simulink model "InverseDynamicsController"  (R2022a)
settings: Solver=VariableStepAuto  StartTime=0.0  StopTime=10.0  RelTol=1e-3
values from neighbouring files (symbols this model uses):
  dt = 0.1    [param.m]    (also in param_10.m; param_7.m)
  F_v = zeros(6,6)    [param.m]    (also in param_10.m; param_7.m)
  K_d = diag([50 50 50 50 50 50])    [param.m]    (also in param_10.m = diag([40 40 40 40 40 40]); param_7.m = diag([40 40 40 40 40 40]))
  K_p = diag([200 200 200 200 200 200])    [param.m]    (also in param_10.m; param_7.m)
  q0 = (ik(T0))'    [param.m]    (also in param_10.m; param_7.m)
settings Model: Creator=niteshkalra  LastModifiedBy=niteshkalra

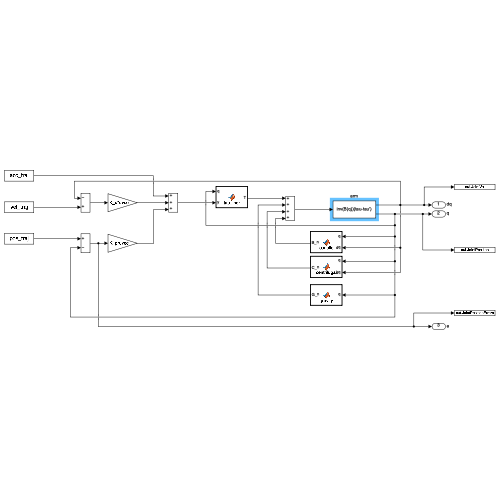
[thumbnail: Simulink's stored preview of the top-level diagram]
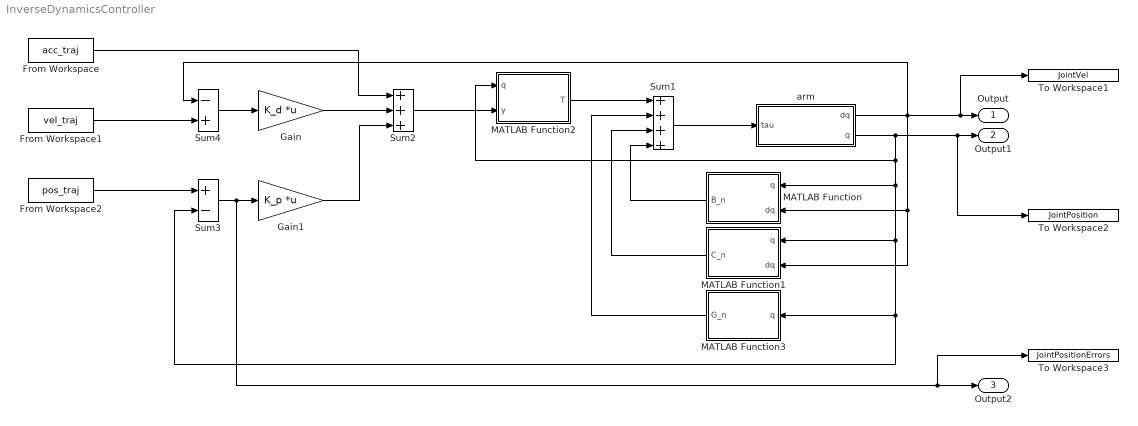
== system InverseDynamicsController ==
  From Workspace : FromWorkspace  VariableName=acc_traj  SampleTime=dt
  From Workspace1 : FromWorkspace  VariableName=vel_traj  SampleTime=dt
  From Workspace2 : FromWorkspace  VariableName=pos_traj  SampleTime=dt
  Gain : Gain  Gain=K_d  Multiplication=Matrix(K*u) (u vector)
  Gain1 : Gain  Gain=K_p  Multiplication=Matrix(K*u) (u vector)
  MATLAB Function : MATLAB Function  TreatAsAtomicUnit=on
  MATLAB Function1 : MATLAB Function  TreatAsAtomicUnit=on
  MATLAB Function2 : MATLAB Function  TreatAsAtomicUnit=on
  MATLAB Function3 : MATLAB Function  TreatAsAtomicUnit=on
  Sum1 : Sum  Inputs=++++
  Sum2 : Sum  Inputs=+++
  Sum3 : Sum  Inputs=+-
  Sum4 : Sum  Inputs=-+
  To Workspace1 : ToWorkspace  VariableName=JointVel  SaveFormat=Timeseries  SampleTime=-1
  To Workspace2 : ToWorkspace  VariableName=JointPosition  SaveFormat=Timeseries  SampleTime=-1
  To Workspace3 : ToWorkspace  VariableName=JointPositionErrors  SaveFormat=Timeseries  SampleTime=-1
  arm : Subsystem
      mask Display: disp('inv(B(q))(tau-tau'')')
  Output : Outport  SignalName=dq
  Output1 : Outport  Port=2  SignalName=q
  Output2 : Outport  Port=3  SignalName=e
  wires:
  MATLAB Function2/1(T) -> Sum1/1
  Sum2/1 -> MATLAB Function2/2(y)
  Gain/1 -> Sum2/2
  Gain1/1 -> Sum2/3
  Sum4/1 -> Gain/1
  From Workspace2/1 -> Sum3/1
  From Workspace/1 -> Sum2/1
  arm/1(dq) -> Sum4/1, MATLAB Function1/2(dq), MATLAB Function/2(dq), To Workspace1/1, Output/1
  arm/2("q ") -> MATLAB Function/1(q), MATLAB Function1/1(q), MATLAB Function3/1(q), Sum3/2, MATLAB Function2/1(q), To Workspace2/1, Output1/1
  Sum3/1 -> To Workspace3/1, Output2/1, Gain1/1
  Sum1/1 -> arm/1(tau)
  MATLAB Function/1(B_n) -> Sum1/4
  MATLAB Function1/1(C_n) -> Sum1/3
  MATLAB Function3/1(G_n) -> Sum1/2
  From Workspace1/1 -> Sum4/2

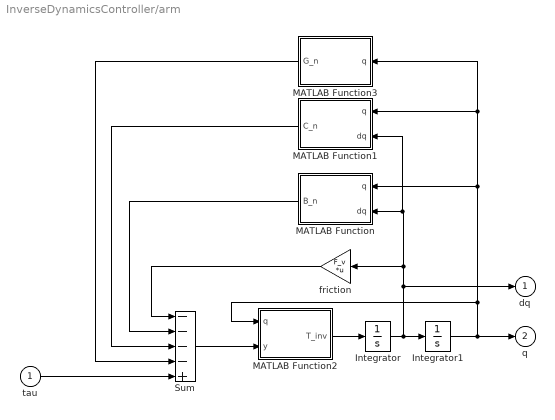
== system InverseDynamicsController/arm ==
  tau : Inport
  Integrator : Integrator  InitialCondition=[0 0 0 0 0 0]'  ZeroCross=off
  Integrator1 : Integrator  InitialCondition=q0  ZeroCross=off
  MATLAB Function : MATLAB Function  TreatAsAtomicUnit=on
  MATLAB Function1 : MATLAB Function  TreatAsAtomicUnit=on
  MATLAB Function2 : MATLAB Function  TreatAsAtomicUnit=on
  MATLAB Function3 : MATLAB Function  TreatAsAtomicUnit=on
  Sum : Sum  Inputs=----+  InputSameDT=on  SaturateOnIntegerOverflow=on  OutDataTypeStr=Inherit: Same as first input
  friction : Gain  Gain=F_v  Multiplication=Matrix(K*u)  SaturateOnIntegerOverflow=on  OutDataTypeStr=Inherit: Same as input  ParamDataTypeStr=Inherit: Same as input
      mask Display: disp('F_v')
  dq : Outport  InitialOutput=0
  "q " : Outport  Port=2  InitialOutput=0
  wires:
  tau/1 -> Sum/5
  Integrator1/1 -> MATLAB Function3/1(q), MATLAB Function1/1(q), MATLAB Function/1(q), MATLAB Function2/1(q), "q "/1
  Integrator/1 -> MATLAB Function1/2(dq), MATLAB Function/2(dq), friction/1, dq/1, Integrator1/1
  Sum/1 -> MATLAB Function2/2(y)
  friction/1 -> Sum/1
  MATLAB Function2/1(T_inv) -> Integrator/1
  MATLAB Function/1(B_n) -> Sum/2
  MATLAB Function1/1(C_n) -> Sum/3
  MATLAB Function3/1(G_n) -> Sum/4

== matlab function InverseDynamicsController/arm/MATLAB Function1 ==
  data: q input; C_n output; dq input
function C_n = centrifugal(q,dq)

% Extracting from input matrices
q1 = q(1);
q2 = q(2);
q3 = q(3);
q4 = q(4);
q5 = q(5);
q6 = q(6);

dq1 = dq(1);
dq2 = dq(2);
dq3 = dq(3);
dq4 = dq(4);
dq5 = dq(5);
dq6 = dq(6);

%Inertia constants in kg.m^2
I1 = 1.43;
I2 = 1.75;
I3 = 1.38;
I4 = 0.69;
I5 = 0.372;
I6 = 0.333;
I7 = 0.298;
I8 = -0.134;
I9 = 0.0238;
I10 = -0.0213;
I11 = -0.0142;
I12 = -0.011;
I13 = -0.00379;
I14 = 0.00164;
I15 = 0.00125;
I16 = 0.00124;
I17 = 0.000642;
I18 = 0.000431;
I19 = 0.0003;
I20 = -0.000202;
I21 = -0.0001;
I22 = -0.000058;
I23 = 0.00004;

Im = [ 1.14 4.71 0.827 0.2 0.179 0.193 ];

% Coriolis matrix elements
b112=2*(-I3*sin(q2)*cos(q2)+I5*cos(q2+q2+q3) +I7*sin(q2+q3)*cos(q2+q3) -I12*sin(q2+q2+q3)-I15*2*sin(q2+q3)*cos(q2+q3)+I16*cos(q2+q2+q3)+I21*sin(q2+q3)*cos(q2+q3)+I22*(1-2*sin(q2+q3)*sin(q2+q3)))+ I10*(1-2*sin(q2+q3)*sin(q2+q3))+I11*(1-2*sin(q2)*sin(q3));

b113=2*(I5*cos(q2)*cos(q2+q3)+I7*sin(q2+q3)*cos(q2+q3)-I12*cos(q2)*sin(q2+q2)+ I15*2*sin(q2+q3)*cos(q2+q3)+I16*cos(q2)*cos(q2+q3)+I21*sin(q2+q3)*cos(q2+q3)+I22*(1-2*sin(q2+q3)*sin(q2+q3)))+I10*(1-2*sin(q2+q3)*sin(q2+q3));

b115=2*(-sin(q2+q3)*cos(q2+q3)+I15*2*sin(q2+q3)*cos(q2+q3)+I16*cos(q2)*cos(q2+q3)+I22*cos(q2+q3)*cos(q2+q3));

b123=2*(-I8*sin(q2+q3)+I13*cos(q2+q3)+I18*sin(q2+q3));

b214=I14*sin(q2+q3)+I19*sin(q2+q3)+2*I20*sin(q2+q3)*(1-0.5);

b223=2*(-I12*sin(q3)+I5*cos(q3)+I16*cos(q3));

b225=2*(I16*cos(q3)+I21);

b235=2*(I16*cos(q3)+I22);

b314=2*(I20*sin(q2+q3)*(1-0.5))+I14*sin(q2+q3)+I19*sin(q2+q3);

b412=-1*(I14*sin(q2+q3)+I19*sin(q2+q3)+2*I20*sin(q2+q3)*(1-0.5));

b412=b214;

b413=-1*(I14*sin(q2+q3)+I19*sin(q2+q3)+2*I20*sin(q2+q3)*(1-0.5));

b413=-1*b314;

b415=-I20*sin(q2+q3)-I17*sin(q2+q3);

b514=I20*sin(q2+q3)+I17*sin(q2+q3);


% Centrifugal matrix elements
c12 = I4*cos(q2)-I8*sin(q2+q3)-I9*sin(q2)+I13*cos(q2+q3)+I18*sin(q2+q3);
c13 = 0.5*b123;
c21 = -0.5*b112;
c23 = 0.5*b223;
c31 = -0.5*b113;
c32 = -1*c23;

c51 = -0.5*b115;
c52 = -0.5*b225;

% %Centrifugal matrix C
% C=zeros(6,6);
% 
% C(1,2) = c12;
% C(1,3) = c13;
% 
% C(2,1) = c21;
% C(2,3) = c23;
% 
% C(3,1) = c31;
% C(3,2) = c32;
% 
% C(5,1) = c51;
% C(5,2) = c52;

% C_n = C.*[qd1^2; qd2^2; qd3^2; 0; 0; 0];

% C_test = [C(1,1), C(1,2), C(1,3);
%     C(2,1), C(2,2), C(2,3);
%     C(3,1), C(3,2), C(3,3)];
% 
% C_n = C_test*[dq1^2; dq2^2; dq3^2];

C_n = [c12*dq2^2 + c13*dq3^2;
    c21*dq1^2 + c23*dq3^2;
    c13*dq1^2 + c32*dq2^2;
    0;
    c51*dq1^2 + c52*dq2^2;
    0];


end

== matlab function InverseDynamicsController/MATLAB Function2 ==
  data: q input; T output; y input
function T = tau_iner(q,y)

% Extracting from input matrix
q1 = q(1);
q2 = q(2);
q3 = q(3);
q4 = q(4);
q5 = q(5);
q6 = q(6);

%Inertia constants in kg.m^2
I1 = 1.43;
I2 = 1.75;
I3 = 1.38;
I4 = 0.69;
I5 = 0.372;
I6 = 0.333;
I7 = 0.298;
I8 = -0.134;
I9 = 0.0238;
I10 = -0.0213;
I11 = -0.0142;
I12 = -0.011;
I13 = -0.00379;
I14 = 0.00164;
I15 = 0.00125;
I16 = 0.00124;
I17 = 0.000642;
I18 = 0.000431;
I19 = 0.0003;
I20 = -0.000202;
I21 = -0.0001;
I22 = -0.000058;
I23 = 0.00004;

Im = [ 1.14 4.71 0.827 0.2 0.179 0.193 ];

% Inertia matrix elements
M11 = Im(1)+I1+(I3*cos(q2)*cos(q2))+(I7*sin(q2+q3)*sin(q2+q3))+(I10*sin(q2+q3)*cos(q2+q3))+(I11*sin(q2)*cos(q2))+(I21*sin(q2+q3)*sin(q2+q3))+2+(I5*cos(q2)*sin(q2+q3))+(I12*cos(q2)*cos(q2+q3))+(I15*sin(q2+q3)*sin(q2+q3))+(I16*cos(q2)*sin(q2+q3))+(I22*sin(q2+q3)*cos(q2+q3));

M12 = (I4*sin(q2))+(I8*cos(q2+q3))+(I9*cos(q2))+(I13*sin(q2+q3))-(I18*cos(q2+q3));

M13 = (I8*cos(q2+q3))+(I13*sin(q2+q3))-(I18*cos(q2+q3));

M22 = Im(2)+I2+I6+2*(I5*sin(q3)+I12*cos(q2)+I15+I16*sin(q3));

M23 = (I5*sin(q3))+I6+(I12*cos(q3))+(I16*sin(q3))+(2*I15);

M33 = Im(3)+I6+(2*I15);

M35 = I15+I17;

M44 = Im(4)+I14;

M55 = Im(5)+I17;

M66 = Im(6)+I23;

M21 = M12;

M31 = M13;

M32 = M23;

%% M Matrix with coupling interactions- Centralized Control

M = [M11 M12 M13 0 0 0;
    M21 M22 M23 0 0 0;
    M31 M32 M33 0 M35 0;
    0 0 0 M44 0 0;
    0 0 0 0 M55 0;
    0 0 0 0 0 M66];

T = M*y;

end

== matlab function InverseDynamicsController/arm/MATLAB Function2 ==
  data: q input; T_inv output; y input
function T_inv = tau_inerinv(q,y)

% Extracting from input matrix
q1 = q(1);
q2 = q(2);
q3 = q(3);
q4 = q(4);
q5 = q(5);
q6 = q(6);

%Inertia constants in kg.m^2
I1 = 1.43;
I2 = 1.75;
I3 = 1.38;
I4 = 0.69;
I5 = 0.372;
I6 = 0.333;
I7 = 0.298;
I8 = -0.134;
I9 = 0.0238;
I10 = -0.0213;
I11 = -0.0142;
I12 = -0.011;
I13 = -0.00379;
I14 = 0.00164;
I15 = 0.00125;
I16 = 0.00124;
I17 = 0.000642;
I18 = 0.000431;
I19 = 0.0003;
I20 = -0.000202;
I21 = -0.0001;
I22 = -0.000058;
I23 = 0.00004;

Im = [ 1.14 4.71 0.827 0.2 0.179 0.193 ];

% Inertia matrix elements
M11 = Im(1)+I1+(I3*cos(q2)*cos(q2))+(I7*sin(q2+q3)*sin(q2+q3))+(I10*sin(q2+q3)*cos(q2+q3))+(I11*sin(q2)*cos(q2))+(I21*sin(q2+q3)*sin(q2+q3))+2+(I5*cos(q2)*sin(q2+q3))+(I12*cos(q2)*cos(q2+q3))+(I15*sin(q2+q3)*sin(q2+q3))+(I16*cos(q2)*sin(q2+q3))+(I22*sin(q2+q3)*cos(q2+q3));

M12 = (I4*sin(q2))+(I8*cos(q2+q3))+(I9*cos(q2))+(I13*sin(q2+q3))-(I18*cos(q2+q3));

M13 = (I8*cos(q2+q3))+(I13*sin(q2+q3))-(I18*cos(q2+q3));

M22 = Im(2)+I2+I6+2*(I5*sin(q3)+I12*cos(q2)+I15+I16*sin(q3));

M23 = (I5*sin(q3))+I6+(I12*cos(q3))+(I16*sin(q3))+(2*I15);

M33 = Im(3)+I6+(2*I15);

M35 = I15+I17;

M44 = Im(4)+I14;

M55 = Im(5)+I17;

M66 = Im(6)+I23;

M21 = M12;

M31 = M13;

M32 = M23;

%% M Matrix with coupling interactions- Centralized Control

M = [M11 M12 M13 0 0 0;
    M21 M22 M23 0 0 0;
    M31 M32 M33 0 M35 0;
    0 0 0 M44 0 0;
    0 0 0 0 M55 0;
    0 0 0 0 0 M66];

T_inv = inv(M)*y;

end

== matlab function InverseDynamicsController/MATLAB Function ==
  data: q input; B_n output; dq input
function B_n = coriolis(q,dq)

% Extracting from input matrices
q1 = q(1);
q2 = q(2);
q3 = q(3);
q4 = q(4);
q5 = q(5);
q6 = q(6);

dq1 = dq(1);
dq2 = dq(2);
dq3 = dq(3);
dq4 = dq(4);
dq5 = dq(5);
dq6 = dq(6);

%Inertia constants in kg.m^2
I1 = 1.43;
I2 = 1.75;
I3 = 1.38;
I4 = 0.69;
I5 = 0.372;
I6 = 0.333;
I7 = 0.298;
I8 = -0.134;
I9 = 0.0238;
I10 = -0.0213;
I11 = -0.0142;
I12 = -0.011;
I13 = -0.00379;
I14 = 0.00164;
I15 = 0.00125;
I16 = 0.00124;
I17 = 0.000642;
I18 = 0.000431;
I19 = 0.0003;
I20 = -0.000202;
I21 = -0.0001;
I22 = -0.000058;
I23 = 0.00004;

Im = [ 1.14 4.71 0.827 0.2 0.179 0.193 ];

% Coriolis matrix elements
b112=2*(-I3*sin(q2)*cos(q2)+I5*cos(q2+q2+q3) +I7*sin(q2+q3)*cos(q2+q3) -I12*sin(q2+q2+q3)-I15*2*sin(q2+q3)*cos(q2+q3)+I16*cos(q2+q2+q3)+I21*sin(q2+q3)*cos(q2+q3)+I22*(1-2*sin(q2+q3)*sin(q2+q3)))+ I10*(1-2*sin(q2+q3)*sin(q2+q3))+I11*(1-2*sin(q2)*sin(q3));

b113=2*(I5*cos(q2)*cos(q2+q3)+I7*sin(q2+q3)*cos(q2+q3)-I12*cos(q2)*sin(q2+q2)+ I15*2*sin(q2+q3)*cos(q2+q3)+I16*cos(q2)*cos(q2+q3)+I21*sin(q2+q3)*cos(q2+q3)+I22*(1-2*sin(q2+q3)*sin(q2+q3)))+I10*(1-2*sin(q2+q3)*sin(q2+q3));

b115=2*(-sin(q2+q3)*cos(q2+q3)+I15*2*sin(q2+q3)*cos(q2+q3)+I16*cos(q2)*cos(q2+q3)+I22*cos(q2+q3)*cos(q2+q3));

b123=2*(-I8*sin(q2+q3)+I13*cos(q2+q3)+I18*sin(q2+q3));

b214=I14*sin(q2+q3)+I19*sin(q2+q3)+2*I20*sin(q2+q3)*(1-0.5);

b223=2*(-I12*sin(q3)+I5*cos(q3)+I16*cos(q3));

b225=2*(I16*cos(q3)+I21);

b235=2*(I16*cos(q3)+I22);

b314=2*(I20*sin(q2+q3)*(1-0.5))+I14*sin(q2+q3)+I19*sin(q2+q3);

b412=-1*(I14*sin(q2+q3)+I19*sin(q2+q3)+2*I20*sin(q2+q3)*(1-0.5));

b412=b214;

b413=-1*(I14*sin(q2+q3)+I19*sin(q2+q3)+2*I20*sin(q2+q3)*(1-0.5));

b413=-1*b314;

b415=-I20*sin(q2+q3)-I17*sin(q2+q3);

b514=I20*sin(q2+q3)+I17*sin(q2+q3);

% Coriolis Matrix B
% B = zeros(15,6);
% 
% B(1,1) = b112;
% B(1,2) = b113;
% B(1,4) = b115;
% B(1,6) = b123;
% 
% B(2,3) = b214;
% B(2,6) = b223;
% B(2,8) = b225;
% B(2,11) = b235;
% 
% B(3,3) = b314;
% 
% B(4,1) = b412;
% B(4,2) = b412;
% B(4,4) = b415;
% 
% B(5,3) = b514;

% B_n = B.*[qd1*qd2; qd1*qd3; qd2*qd3; 0; 0; 0];

% B_test = [B(1,1) B(1,2) B(1,3);
%     B(2,1) B(2,2) B(2,3);
%     B(3,1) B(3,2) B(3,3)];
% 
% B_n = B_test*[dq1*dq2; dq1*dq3; dq2*dq3];

B_n = [b112*dq1*dq2 + b113*dq1*dq3 + b123*dq2*dq3;
    b223*dq2*dq3;
    0;
    b412*dq1*dq2 + b413*dq1*dq3;
    0;
    0];


end

== matlab function InverseDynamicsController/arm/MATLAB Function ==
  data: q input; B_n output; dq input
function B_n = coriolis(q,dq)

% Extracting from input matrices
q1 = q(1);
q2 = q(2);
q3 = q(3);
q4 = q(4);
q5 = q(5);
q6 = q(6);

dq1 = dq(1);
dq2 = dq(2);
dq3 = dq(3);
dq4 = dq(4);
dq5 = dq(5);
dq6 = dq(6);

%Inertia constants in kg.m^2
I1 = 1.43;
I2 = 1.75;
I3 = 1.38;
I4 = 0.69;
I5 = 0.372;
I6 = 0.333;
I7 = 0.298;
I8 = -0.134;
I9 = 0.0238;
I10 = -0.0213;
I11 = -0.0142;
I12 = -0.011;
I13 = -0.00379;
I14 = 0.00164;
I15 = 0.00125;
I16 = 0.00124;
I17 = 0.000642;
I18 = 0.000431;
I19 = 0.0003;
I20 = -0.000202;
I21 = -0.0001;
I22 = -0.000058;
I23 = 0.00004;

Im = [ 1.14 4.71 0.827 0.2 0.179 0.193 ];

% Coriolis matrix elements
b112=2*(-I3*sin(q2)*cos(q2)+I5*cos(q2+q2+q3) +I7*sin(q2+q3)*cos(q2+q3) -I12*sin(q2+q2+q3)-I15*2*sin(q2+q3)*cos(q2+q3)+I16*cos(q2+q2+q3)+I21*sin(q2+q3)*cos(q2+q3)+I22*(1-2*sin(q2+q3)*sin(q2+q3)))+ I10*(1-2*sin(q2+q3)*sin(q2+q3))+I11*(1-2*sin(q2)*sin(q3));

b113=2*(I5*cos(q2)*cos(q2+q3)+I7*sin(q2+q3)*cos(q2+q3)-I12*cos(q2)*sin(q2+q2)+ I15*2*sin(q2+q3)*cos(q2+q3)+I16*cos(q2)*cos(q2+q3)+I21*sin(q2+q3)*cos(q2+q3)+I22*(1-2*sin(q2+q3)*sin(q2+q3)))+I10*(1-2*sin(q2+q3)*sin(q2+q3));

b115=2*(-sin(q2+q3)*cos(q2+q3)+I15*2*sin(q2+q3)*cos(q2+q3)+I16*cos(q2)*cos(q2+q3)+I22*cos(q2+q3)*cos(q2+q3));

b123=2*(-I8*sin(q2+q3)+I13*cos(q2+q3)+I18*sin(q2+q3));

b214=I14*sin(q2+q3)+I19*sin(q2+q3)+2*I20*sin(q2+q3)*(1-0.5);

b223=2*(-I12*sin(q3)+I5*cos(q3)+I16*cos(q3));

b225=2*(I16*cos(q3)+I21);

b235=2*(I16*cos(q3)+I22);

b314=2*(I20*sin(q2+q3)*(1-0.5))+I14*sin(q2+q3)+I19*sin(q2+q3);

b412=-1*(I14*sin(q2+q3)+I19*sin(q2+q3)+2*I20*sin(q2+q3)*(1-0.5));

b412=b214;

b413=-1*(I14*sin(q2+q3)+I19*sin(q2+q3)+2*I20*sin(q2+q3)*(1-0.5));

b413=-1*b314;

b415=-I20*sin(q2+q3)-I17*sin(q2+q3);

b514=I20*sin(q2+q3)+I17*sin(q2+q3);

% Coriolis Matrix B
% B = zeros(15,6);
% 
% B(1,1) = b112;
% B(1,2) = b113;
% B(1,4) = b115;
% B(1,6) = b123;
% 
% B(2,3) = b214;
% B(2,6) = b223;
% B(2,8) = b225;
% B(2,11) = b235;
% 
% B(3,3) = b314;
% 
% B(4,1) = b412;
% B(4,2) = b412;
% B(4,4) = b415;
% 
% B(5,3) = b514;

% B_n = B.*[qd1*qd2; qd1*qd3; qd2*qd3; 0; 0; 0];

% B_test = [B(1,1) B(1,2) B(1,3);
%     B(2,1) B(2,2) B(2,3);
%     B(3,1) B(3,2) B(3,3)];
% 
% B_n = B_test*[dq1*dq2; dq1*dq3; dq2*dq3];

B_n = [b112*dq1*dq2 + b113*dq1*dq3 + b123*dq2*dq3;
    b223*dq2*dq3;
    0;
    b412*dq1*dq2 + b413*dq1*dq3;
    0;
    0];


end

== matlab function InverseDynamicsController/MATLAB Function3 ==
  data: q input; G_n output
function G_n = gravity(q)

% Extracting from input matrices
q1 = q(1);
q2 = q(2);
q3 = q(3);
q4 = q(4);
q5 = q(5);
q6 = q(6);

% Gravitational constants (N.m)
g1 = -37.2;
g2 = -8.44;
g3 = 1.02;
g4 = 0.249;
g5 = -0.0282;

% Gravity matrix elements
G2 = (g1*cos(q1))+(g2*sin(q2+q3))+(g3*sin(q2))+(g4*cos(q2+q3))+(g5*sin(q2+q3));
G3 = (g2*sin(q2+q3))+(g4*cos(q2+q3))+(g5*sin(q2+q3));
G5 = g5*sin(q2+q3);

% Gravity matrix G

G_n = [0; G2; G3; 0; G5; 0];

end

== matlab function InverseDynamicsController/arm/MATLAB Function3 ==
  data: q input; G_n output
function G_n = gravity(q)

% Extracting from input matrices
q1 = q(1);
q2 = q(2);
q3 = q(3);
q4 = q(4);
q5 = q(5);
q6 = q(6);

% Gravitational constants (N.m)
g1 = -37.2;
g2 = -8.44;
g3 = 1.02;
g4 = 0.249;
g5 = -0.0282;

% Gravity matrix elements
G2 = (g1*cos(q1))+(g2*sin(q2+q3))+(g3*sin(q2))+(g4*cos(q2+q3))+(g5*sin(q2+q3));
G3 = (g2*sin(q2+q3))+(g4*cos(q2+q3))+(g5*sin(q2+q3));
G5 = g5*sin(q2+q3);

% Gravity matrix G

G_n = [0; G2; G3; 0; G5; 0];

end

== matlab function InverseDynamicsController/MATLAB Function1 ==
  data: q input; C_n output; dq input
function C_n = centrifugal(q,dq)

% Extracting from input matrices
q1 = q(1);
q2 = q(2);
q3 = q(3);
q4 = q(4);
q5 = q(5);
q6 = q(6);

dq1 = dq(1);
dq2 = dq(2);
dq3 = dq(3);
dq4 = dq(4);
dq5 = dq(5);
dq6 = dq(6);

%Inertia constants in kg.m^2
I1 = 1.43;
I2 = 1.75;
I3 = 1.38;
I4 = 0.69;
I5 = 0.372;
I6 = 0.333;
I7 = 0.298;
I8 = -0.134;
I9 = 0.0238;
I10 = -0.0213;
I11 = -0.0142;
I12 = -0.011;
I13 = -0.00379;
I14 = 0.00164;
I15 = 0.00125;
I16 = 0.00124;
I17 = 0.000642;
I18 = 0.000431;
I19 = 0.0003;
I20 = -0.000202;
I21 = -0.0001;
I22 = -0.000058;
I23 = 0.00004;

Im = [ 1.14 4.71 0.827 0.2 0.179 0.193 ];

% Coriolis matrix elements
b112=2*(-I3*sin(q2)*cos(q2)+I5*cos(q2+q2+q3) +I7*sin(q2+q3)*cos(q2+q3) -I12*sin(q2+q2+q3)-I15*2*sin(q2+q3)*cos(q2+q3)+I16*cos(q2+q2+q3)+I21*sin(q2+q3)*cos(q2+q3)+I22*(1-2*sin(q2+q3)*sin(q2+q3)))+ I10*(1-2*sin(q2+q3)*sin(q2+q3))+I11*(1-2*sin(q2)*sin(q3));

b113=2*(I5*cos(q2)*cos(q2+q3)+I7*sin(q2+q3)*cos(q2+q3)-I12*cos(q2)*sin(q2+q2)+ I15*2*sin(q2+q3)*cos(q2+q3)+I16*cos(q2)*cos(q2+q3)+I21*sin(q2+q3)*cos(q2+q3)+I22*(1-2*sin(q2+q3)*sin(q2+q3)))+I10*(1-2*sin(q2+q3)*sin(q2+q3));

b115=2*(-sin(q2+q3)*cos(q2+q3)+I15*2*sin(q2+q3)*cos(q2+q3)+I16*cos(q2)*cos(q2+q3)+I22*cos(q2+q3)*cos(q2+q3));

b123=2*(-I8*sin(q2+q3)+I13*cos(q2+q3)+I18*sin(q2+q3));

b214=I14*sin(q2+q3)+I19*sin(q2+q3)+2*I20*sin(q2+q3)*(1-0.5);

b223=2*(-I12*sin(q3)+I5*cos(q3)+I16*cos(q3));

b225=2*(I16*cos(q3)+I21);

b235=2*(I16*cos(q3)+I22);

b314=2*(I20*sin(q2+q3)*(1-0.5))+I14*sin(q2+q3)+I19*sin(q2+q3);

b412=-1*(I14*sin(q2+q3)+I19*sin(q2+q3)+2*I20*sin(q2+q3)*(1-0.5));

b412=b214;

b413=-1*(I14*sin(q2+q3)+I19*sin(q2+q3)+2*I20*sin(q2+q3)*(1-0.5));

b413=-1*b314;

b415=-I20*sin(q2+q3)-I17*sin(q2+q3);

b514=I20*sin(q2+q3)+I17*sin(q2+q3);


% Centrifugal matrix elements
c12 = I4*cos(q2)-I8*sin(q2+q3)-I9*sin(q2)+I13*cos(q2+q3)+I18*sin(q2+q3);
c13 = 0.5*b123;
c21 = -0.5*b112;
c23 = 0.5*b223;
c31 = -0.5*b113;
c32 = -1*c23;

c51 = -0.5*b115;
c52 = -0.5*b225;

% %Centrifugal matrix C
% C=zeros(6,6);
% 
% C(1,2) = c12;
% C(1,3) = c13;
% 
% C(2,1) = c21;
% C(2,3) = c23;
% 
% C(3,1) = c31;
% C(3,2) = c32;
% 
% C(5,1) = c51;
% C(5,2) = c52;

% C_n = C.*[qd1^2; qd2^2; qd3^2; 0; 0; 0];

% C_test = [C(1,1), C(1,2), C(1,3);
%     C(2,1), C(2,2), C(2,3);
%     C(3,1), C(3,2), C(3,3)];
% 
% C_n = C_test*[dq1^2; dq2^2; dq3^2];

C_n = [c12*dq2^2 + c13*dq3^2;
    c21*dq1^2 + c23*dq3^2;
    c13*dq1^2 + c32*dq2^2;
    0;
    c51*dq1^2 + c52*dq2^2;
    0];


end
